simulink model "playback_data"  (R2015a)
settings: Solver=FixedStepDiscrete  SolverMode=SingleTasking  StartTime=76  StopTime=110  FixedStep=sample_time  RelTol=1e-3
undefined symbols (not defined in the file): A1_notch_f1, A2_notch_f1, A_kalman_swing_load, A_kalman_transverse, A_kalman_vertical, A_lpf_accelerometer, A_lpf_dtau, A_lpf_fourbar_angles, A_lpf_imu, A_lpf_lateral_angle, B1_lpf_accelerometer, B1_lpf_dtau, B1_lpf_fourbar_angles, B1_lpf_imu, B1_lpf_lateral_angle, B1_notch_f1, B2_lpf_accelerometer, B2_lpf_dtau, B2_lpf_fourbar_angles, B2_lpf_imu, B2_lpf_lateral_angle, B2_notch_f1, B_dx_versus_x0, B_kalman_swing_load, B_kalman_transverse, B_kalman_vertical, backwards_K_sag_of_t, backwards_P_sag_of_t, C_kalman_swing_load, C_kalman_transverse, C_kalman_vertical, com_leg_motor, com_torso, contact_threshold, control_start_time, d_ankle_to_foot, d_vertical_com, desired_com_forward_velocity, desired_com_lateral_velocity, desired_initial_leg_roll_left, desired_initial_leg_roll_right, desired_stance_beta2, desired_standing_torso_pitch, desired_standing_torso_roll, desired_standing_z, desired_torso_pitch, desired_torso_roll, Discrete, enable_bouncing, fcut_contact, fdesignblkfcn, forward_dx_of_dxstar, forward_x_of_dxstar, g, gcbh, HIP_MTR_MAX_CONT_TORQUE, HIP_MTR_MAX_TORQUE, i_leg_motor, i_robot, i_torso ... (+78)
libraries: simulink x65, dsparch4 x18, ctrlSharedLib x14, dspfdesign x4
(part 1 of 13)
settings Model: CovSFcnEnable=off  Creator=wmartin  LastModifiedBy=wmartin
settings SolverCC: EnableConcurrentExecution=on
settings DataIOCC: LimitDataPoints=off  MaxDataPoints=1000000000  SaveFormat=StructureWithTime  SignalLogging=off  DSMLogging=off  VisualizeSimOutput=off
settings OptimizationCC: BlockReduction=off  OptimizeBlockIOStorage=off  BufferReuse=off  GlobalBufferReuse=off  ExpressionFolding=off  ExpressionDepthLimit=2147483647  LocalBlockOutputs=off  SimCompilerOptimization=on
settings DebuggingCC: UnderspecifiedInitializationDetection=Classic  MergeDetectMultiDrivingBlocksExec=none  SolverPrmCheckMsg=warning  StateNameClashWarn=warning
settings HardwareCC: ProdIntDivRoundTo=Zero  ProdEndianess=LittleEndian  ProdLongLongMode=on  ProdHWDeviceType=Generic->32-bit x86 compatible
settings ModelReferenceCC: UpdateModelReferenceTargets=IfOutOfDate  ModelReferenceNumInstancesAllowed=Single  ModelReferenceMinAlgLoopOccurrences=on
settings RTWCC: SystemTargetFile=slrt.tlc  TemplateMakefile=slrt_default_tmf  Description=Simulink Real-Time  RTWVerbose=off  RTWCompilerOptimization=on
settings CodeAppCC: MaxIdLength=256
settings TargetCC: CodeReplacementLibrary=XPC_BLAS  ParMdlRefBuildCompliant=on  ConcurrentExecutionCompliant=on  MatFileLogging=on  MATLABClassNameForMDSCustomization=xpcAperiodicCustomization

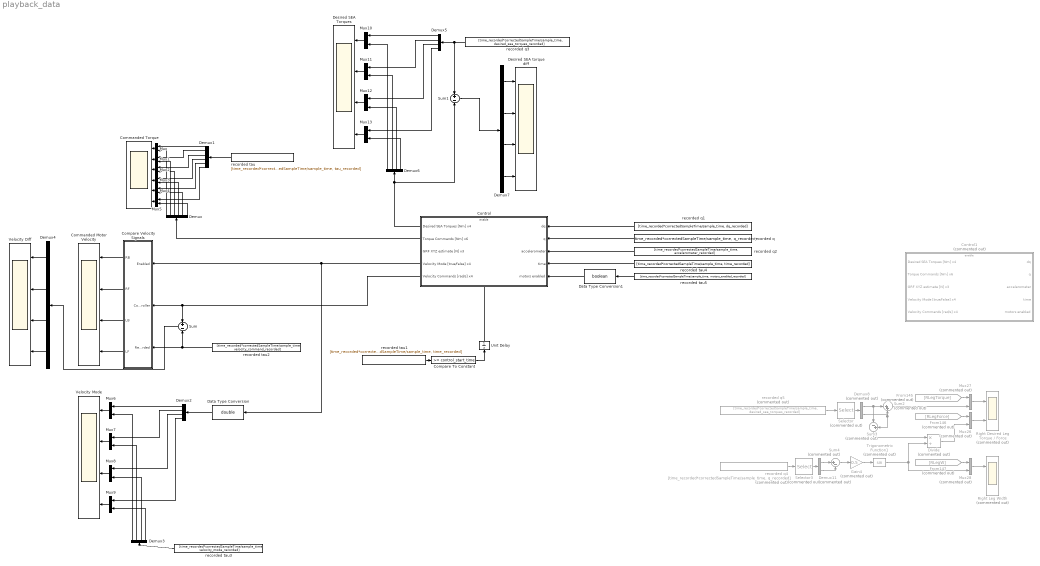
== system playback_data ==
  Commanded Motor Velocity : Scope  NumInputPorts=4
      settings: YMin=-0.45~-1~-1~-1  YMax=0.35~1~1~1  SaveName=SeaTorques  SampleInput=on  SampleTime=sample_time
  Commanded Torque : Scope  NumInputPorts=6
      settings: TimeRange=75  YMin=-75~-150~31~-1~-1~12.5  YMax=125~50~44~1~1~37.5  SampleInput=on
  Compare To Constant : simulink/Logic and Bit Operations/Compare To Constant  relop=>=  const=control_start_time  OutDataTypeStr=boolean
  Compare Velocity Signals : Subsystem
  Control : Subsystem
  Control1 : Subsystem  Commented=on
  Data Type Conversion : DataTypeConversion  OutDataTypeStr=double
  Data Type Conversion1 : DataTypeConversion  OutDataTypeStr=boolean
  Demux : Demux  Outputs=6
  Demux1 : Demux  Outputs=6
  Demux11 : Demux  Commented=on  Outputs=2
  Demux{2..7} (6 alike) : Demux
  Demux8 : Demux  Commented=on  Outputs=2
  Desired SEA Torques : Scope  NumInputPorts=4
      settings: YMin=-1~-1~-225~0  YMax=1~1~0~225  SaveName=SeaTorques3  SampleInput=on  SampleTime=sample_time
  Desired SEA torque diff : Scope  NumInputPorts=4
      settings: TimeRange=17.014  YMin=-1~-1~-0.35~-0.35  YMax=1~1~0.35~0.35  SaveName=SeaTorques4  SampleInput=on
  Divide : Product  Commented=on  Inputs=*/
  From145 : From  Commented=on  GotoTag=RLegTorque
  From146 : From  Commented=on  GotoTag=RLegForce
  From147 : From  Commented=on  GotoTag=RLegW
  Gain4 : Gain  Commented=on  Gain=0.5
  Mux{,1..13} (14 alike) : Mux  Inputs=2
  Mux26 : Mux  Commented=on  Inputs=2
  Mux27 : Mux  Commented=on  Inputs=2
  Mux28 : Mux  Commented=on  Inputs=2
  Right Desired Leg Torque / Force : Scope  Commented=on  NumInputPorts=2
      settings: YMin=0~-150  YMax=90~850  SaveName=ScopeData25  SampleInput=on
  Right Leg Width : Scope  Commented=on  NumInputPorts=2
      settings: YMin=0.57~-1  YMax=0.7~1  SaveName=ScopeData26  SampleInput=on
  Selector : Selector  Commented=on  InputPortWidth=4  Indices=[1 2]
  Selector3 : Selector  Commented=on  InputPortWidth=13  Indices=[1 3]
  Sum : Sum  Inputs=+-
  Sum1 : Sum  Inputs=+-
  Sum2 : Sum  Commented=on  Inputs=|++
  Sum3 : Sum  Commented=on  Inputs=|-+
  Sum4 : Sum  Commented=on  Inputs=|+-
  Trigonometric Function1 : Trigonometry  Commented=on
  Unit Delay : UnitDelay  SampleTime=-1
  Velocity Diff : Scope  NumInputPorts=4
      settings: YMin=-2~-2.5~-3~-4  YMax=2~2.5~3.5~2.5  SaveName=SeaTorques2  SampleInput=on
  Velocity Mode : Scope  NumInputPorts=4
      settings: YMin=1~1~-1~-1  YMax=1~1~1~1  SaveName=SeaTorques1  SampleInput=on  SampleTime=sample_time
  recorded q : FromWorkspace  VariableName=[time_recorded*correctedSampleTime/sample_time, q_recorded]  OutDataTypeStr=double  SampleTime=sample_time  OutputAfterFinalValue=Holding final value
  recorded q1 : FromWorkspace  VariableName=[time_recorded*correctedSampleTime/sample_time, dq_recorded]  OutDataTypeStr=double  SampleTime=sample_time  OutputAfterFinalValue=Holding final value
  recorded q2 : FromWorkspace  VariableName=[time_recorded*correctedSampleTime/sample_time, accelerometer_recorded]  OutDataTypeStr=double  SampleTime=sample_time  OutputAfterFinalValue=Holding final value
  recorded q3 : FromWorkspace  VariableName=[time_recorded*correctedSampleTime/sample_time, desired_sea_torques_recorded]  OutDataTypeStr=double  SampleTime=sample_time  OutputAfterFinalValue=Holding final value
  recorded q4 : FromWorkspace  Commented=on  VariableName=[time_recorded*correctedSampleTime/sample_time, q_recorded]  OutDataTypeStr=double  SampleTime=sample_time  OutputAfterFinalValue=Holding final value
  recorded q5 : FromWorkspace  Commented=on  VariableName=[time_recorded*correctedSampleTime/sample_time, desired_sea_torques_recorded]  OutDataTypeStr=double  SampleTime=sample_time  OutputAfterFinalValue=Holding final value
  recorded tau : FromWorkspace  VariableName=[time_recorded*correctedSampleTime/sample_time, tau_recorded]  OutDataTypeStr=double  SampleTime=sample_time  Interpolate=off  OutputAfterFinalValue=Holding final value
  recorded tau1 : FromWorkspace  VariableName=[time_recorded*correctedSampleTime/sample_time, time_recorded]  OutDataTypeStr=double  SampleTime=sample_time  OutputAfterFinalValue=Holding final value
  recorded tau2 : FromWorkspace  VariableName=[time_recorded*correctedSampleTime/sample_time, velocity_command_recorded]  OutDataTypeStr=double  SampleTime=sample_time  Interpolate=off  OutputAfterFinalValue=Holding final value
  recorded tau3 : FromWorkspace  VariableName=[time_recorded*correctedSampleTime/sample_time, velocity_mode_recorded]  OutDataTypeStr=double  SampleTime=sample_time  Interpolate=off  OutputAfterFinalValue=Holding final value
  recorded tau4 : FromWorkspace  VariableName=[time_recorded*correctedSampleTime/sample_time, time_recorded]  OutDataTypeStr=double  SampleTime=sample_time  OutputAfterFinalValue=Holding final value
  recorded tau5 : FromWorkspace  VariableName=[time_recorded*correctedSampleTime/sample_time, motors_enabled_recorded]  OutDataTypeStr=double  SampleTime=sample_time  OutputAfterFinalValue=Holding final value
  wires:
  recorded tau1/1 -> Compare To Constant/1
  Compare To Constant/1 -> Unit Delay/1
  Unit Delay/1 -> Control/Enable
  Control/2(Torque Commands [Nm] x6) -> Demux/1
  recorded tau/1 -> Demux1/1
  Mux/1 -> Commanded Torque/1
  Mux1/1 -> Commanded Torque/2
  Mux2/1 -> Commanded Torque/3
  Mux3/1 -> Commanded Torque/4
  Mux4/1 -> Commanded Torque/5
  Mux5/1 -> Commanded Torque/6
  Demux1/1 -> Mux/1
  Demux/1 -> Mux/2
  Demux1/2 -> Mux1/1
  Demux1/3 -> Mux2/1
  Demux1/4 -> Mux3/1
  Demux1/5 -> Mux4/1
  Demux1/6 -> Mux5/1
  Demux/2 -> Mux1/2
  Demux/3 -> Mux2/2
  Demux/4 -> Mux3/2
  Demux/5 -> Mux4/2
  Demux/6 -> Mux5/2
  Compare Velocity Signals/1(RB) -> Commanded Motor Velocity/1
  Compare Velocity Signals/2(RF) -> Commanded Motor Velocity/2
  Compare Velocity Signals/3(LB) -> Commanded Motor Velocity/3
  Compare Velocity Signals/4(LF) -> Commanded Motor Velocity/4
  Control/4(Velocity Mode [true/false] x4) -> Data Type Conversion/1, Compare Velocity Signals/1(Enabled)
  recorded tau2/1 -> Sum/2, Compare Velocity Signals/3(Recorded)
  Mux6/1 -> Velocity Mode/1
  Mux7/1 -> Velocity Mode/2
  Mux8/1 -> Velocity Mode/3
  Mux9/1 -> Velocity Mode/4
  Demux2/2 -> Mux7/1
  Demux2/3 -> Mux8/1
  Demux2/4 -> Mux9/1
  recorded tau3/1 -> Demux3/1
  Demux3/1 -> Mux6/2
  Demux3/2 -> Mux7/2
  Demux3/3 -> Mux8/2
  Demux3/4 -> Mux9/2
  Data Type Conversion/1 -> Demux2/1
  Demux2/1 -> Mux6/1
  Control/5(Velocity Commands [rad/s] x4) -> Sum/1, Compare Velocity Signals/2(Controller)
  Sum/1 -> Demux4/1
  Demux4/4 -> Velocity Diff/4
  Demux4/3 -> Velocity Diff/3
  Demux4/2 -> Velocity Diff/2
  Demux4/1 -> Velocity Diff/1
  Mux10/1 -> Desired SEA Torques/1
  Mux11/1 -> Desired SEA Torques/2
  Mux12/1 -> Desired SEA Torques/3
  Mux13/1 -> Desired SEA Torques/4
  Demux5/2 -> Mux11/1
  Demux5/3 -> Mux12/1
  Demux5/4 -> Mux13/1
  Demux6/1 -> Mux10/2
  Demux6/2 -> Mux11/2
  Demux6/3 -> Mux12/2
  Demux6/4 -> Mux13/2
  recorded q3/1 -> Demux5/1, Sum1/1
  Demux5/1 -> Mux10/1
  Control/1(Desired SEA Torques [Nm] x4) -> Sum1/2, Demux6/1
  Demux7/3 -> Desired SEA torque diff/3
  Demux7/2 -> Desired SEA torque diff/2
  Demux7/1 -> Desired SEA torque diff/1
  Demux7/4 -> Desired SEA torque diff/4
  Sum1/1 -> Demux7/1
  recorded q5/1 -> Selector/1
  Selector/1 -> Demux8/1
  Demux8/1 -> Sum3/1, Sum2/1
  Demux8/2 -> Sum3/2, Sum2/2
  Sum2/1 -> Mux27/2
  Sum3/1 -> Divide/1
  Mux27/1 -> Right Desired Leg Torque / Force/1
  Mux26/1 -> Right Desired Leg Torque / Force/2
  From146/1 -> Mux26/1
  From145/1 -> Mux27/1
  recorded q4/1 -> Selector3/1
  Selector3/1 -> Demux11/1
  Demux11/1 -> Sum4/1
  Demux11/2 -> Sum4/2
  Sum4/1 -> Gain4/1
  Gain4/1 -> Trigonometric Function1/1
  Trigonometric Function1/1 -> Divide/2, Mux28/2
  Divide/1 -> Mux26/2
  Mux28/1 -> Right Leg Width/1
  From147/1 -> Mux28/1
  recorded q1/1 -> Control/1(dq)
  recorded q/1 -> Control/2(q)
  recorded q2/1 -> Control/3(accelerometer)
  recorded tau4/1 -> Control/4(time)
  Data Type Conversion1/1 -> Control/5(motors enabled)
  recorded tau5/1 -> Data Type Conversion1/1

== system playback_data/Compare Velocity Signals ==
  Enabled : Inport
  Controller : Inport  Port=2
  Recorded : Inport  Port=3
  Demux : Demux
  Demux1 : Demux
  Demux2 : Demux
  Mux{6..9} (4 alike) : Mux  Inputs=2
  Product{,1..3} (4 alike) : Product
  RB : Outport
  RF : Outport  Port=2
  LB : Outport  Port=3
  LF : Outport  Port=4
  wires:
  Demux/3 -> Mux8/1
  Demux/2 -> Mux7/1
  Demux1/1 -> Mux6/2
  Demux/1 -> Mux6/1
  Product/1 -> RB/1
  Demux/4 -> Mux9/1
  Mux6/1 -> Product/2
  Demux1/4 -> Mux9/2
  Mux7/1 -> Product1/2
  Mux9/1 -> Product3/2
  Recorded/1 -> Demux1/1
  Demux2/3 -> Product2/1
  Demux1/2 -> Mux7/2
  Controller/1 -> Demux/1
  Demux2/1 -> Product/1
  Product3/1 -> LF/1
  Product1/1 -> RF/1
  Product2/1 -> LB/1
  Mux8/1 -> Product2/2
  Demux1/3 -> Mux8/2
  Enabled/1 -> Demux2/1
  Demux2/4 -> Product3/1
  Demux2/2 -> Product1/1

== system playback_data/Control ==
  dq : Inport
  q : Inport  Port=2
  accelerometer : Inport  Port=3
  time : Inport  Port=4
  motors enabled : Inport  Port=5
  Enable : EnablePort  StatesWhenEnabling=reset  PropagateVarSize=During execution  ShowOutputPort=on
  Actuator Control : ModelReference  ModelNameDialog=actuator_control  SimulationMode=Normal  ModelReferenceVersion=1.1246  CopyOfModelName=actuator_control  DefaultDataLogging=on
  Actuator Control with Torque SEA commands : Subsystem  Commented=on
  Behavior Control : Subsystem
  Compute Body Frame Accelerations : Subsystem
  Detect Change : simulink/Logic and Bit Operations/Detect Change  vinit=0  InputProcessing=Inherited  OutDataTypeStr=boolean
  Filter Velocities : Subsystem
  Mux : Mux
  Desired SEA Torques [Nm] x4 : Outport  InitialOutput=[0 0 0 0]
  Torque Commands [Nm] x6 : Outport  Port=2  InitialOutput=[0 0 0 0 0 0]
  GRF XYZ estimate [N] x3 : Outport  Port=3  InitialOutput=[0 0 0]
  Velocity Mode [true/false] x4 : Outport  Port=4  InitialOutput=[false false false false]
  Velocity Commands [rad/s] x4 : Outport  Port=5  InitialOutput=[0 0 0 0]
  wires:
  q/1 -> Behavior Control/4(q), Actuator Control/6
  Actuator Control/1 -> Torque Commands [Nm] x6/1
  Behavior Control/4(GRF XYZ estimates [N N N]) -> GRF XYZ estimate [N] x3/1
  Filter Velocities/1(filtered dq) -> Behavior Control/3(dq)
  dq/1 -> Filter Velocities/1(raw dq), Actuator Control/7
  Actuator Control/2 -> Velocity Mode [true/false] x4/1
  Actuator Control/3 -> Velocity Commands [rad/s] x4/1
  accelerometer/1 -> Compute Body Frame Accelerations/1(accelerometer [g] x3)
  Compute Body Frame Accelerations/1(accelerations [m/s^2] x3) -> Behavior Control/2(Body XYZ Acceleration [m/s^2] x3)
  Enable/1 -> Behavior Control/1(Enabled [true/false])
  Actuator Control/4 -> Desired SEA Torques [Nm] x4/1
  Mux/1 -> Actuator Control/1
  motors enabled/1 -> Detect Change/1
  Detect Change/1 -> Mux/4, Mux/3, Mux/2, Mux/1
  time/1 -> Behavior Control/5(time), Actuator Control/5
  Behavior Control/3(Stance / Swing Control [1/0] x4) -> Actuator Control/4
  Behavior Control/2(Velocity Commands [rad/s] x4) -> Actuator Control/3
  Behavior Control/1(Torque Commands [Nm] x6) -> Actuator Control/2

== system playback_data/Control1 ==
  dq : Inport
  q : Inport  Port=2
  accelerometer : Inport  Port=3
  time : Inport  Port=4
  motors enabled : Inport  Port=5
  Enable : EnablePort  StatesWhenEnabling=reset  PropagateVarSize=During execution  ShowOutputPort=on
  Actuator Control : ModelReference  ModelNameDialog=actuator_control  SimulationMode=Normal  ModelReferenceVersion=1.1246  CopyOfModelName=actuator_control  DefaultDataLogging=on
  Actuator Control with Torque SEA commands : Subsystem  Commented=on
  Behavior Control : Subsystem
  Compute Body Frame Accelerations : Subsystem
  Detect Change : simulink/Logic and Bit Operations/Detect Change  vinit=0  InputProcessing=Inherited  OutDataTypeStr=boolean
  Filter Velocities : Subsystem
  Mux : Mux
  Desired SEA Torques [Nm] x4 : Outport  InitialOutput=[0 0 0 0]
  Torque Commands [Nm] x6 : Outport  Port=2  InitialOutput=[0 0 0 0 0 0]
  GRF XYZ estimate [N] x3 : Outport  Port=3  InitialOutput=[0 0 0]
  Velocity Mode [true/false] x4 : Outport  Port=4  InitialOutput=[false false false false]
  Velocity Commands [rad/s] x4 : Outport  Port=5  InitialOutput=[0 0 0 0]
  wires:
  q/1 -> Behavior Control/4(q), Actuator Control/6
  Actuator Control/1 -> Torque Commands [Nm] x6/1
  Behavior Control/4(GRF XYZ estimates [N N N]) -> GRF XYZ estimate [N] x3/1
  Filter Velocities/1(filtered dq) -> Behavior Control/3(dq)
  dq/1 -> Filter Velocities/1(raw dq), Actuator Control/7
  Actuator Control/2 -> Velocity Mode [true/false] x4/1
  Actuator Control/3 -> Velocity Commands [rad/s] x4/1
  accelerometer/1 -> Compute Body Frame Accelerations/1(accelerometer [g] x3)
  Compute Body Frame Accelerations/1(accelerations [m/s^2] x3) -> Behavior Control/2(Body XYZ Acceleration [m/s^2] x3)
  Enable/1 -> Behavior Control/1(Enabled [true/false])
  Actuator Control/4 -> Desired SEA Torques [Nm] x4/1
  Mux/1 -> Actuator Control/1
  motors enabled/1 -> Detect Change/1
  Detect Change/1 -> Mux/4, Mux/3, Mux/2, Mux/1
  time/1 -> Behavior Control/5(time), Actuator Control/5
  Behavior Control/3(Stance / Swing Control [1/0] x4) -> Actuator Control/4
  Behavior Control/2(Velocity Commands [rad/s] x4) -> Actuator Control/3
  Behavior Control/1(Torque Commands [Nm] x6) -> Actuator Control/2

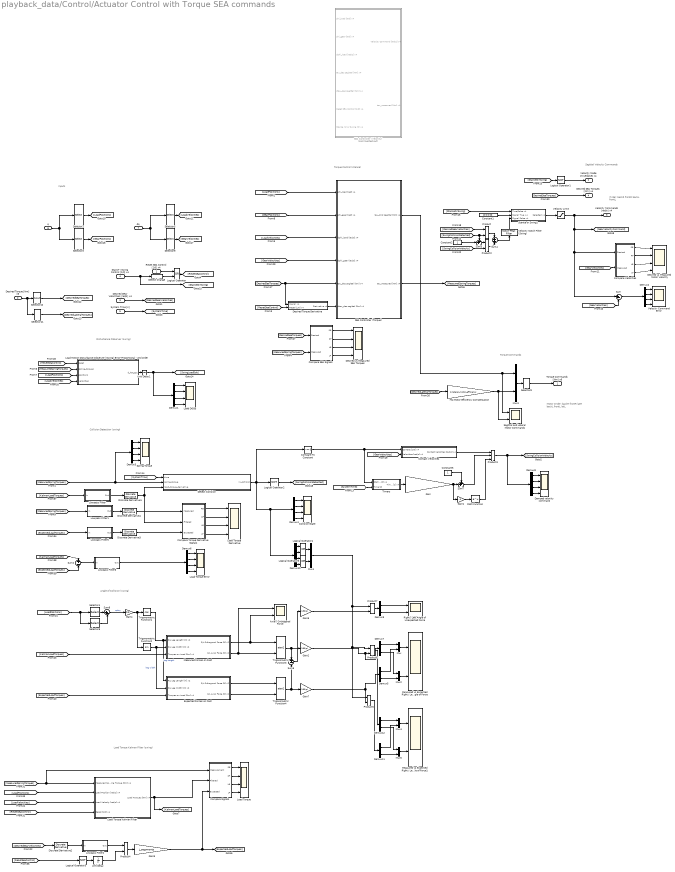
== system playback_data/Control/Actuator Control with Torque SEA commands ==
  note: Order:
      | backR
      | frontR
      | backL
      | frontL
  note: Motor Order:
      |
      | backR
      | frontR
      | latR
      | backL
      | frontL
      | latL
  note: Torque Control (stance)
  note: Inputs
  note: Disturbance Observer (swing)
  note: Torque Commands
  note: Sagittal Velocity Commands
  note: Collision Detection (swing)
  note: Load Torque Kalman Filter (swing)
  note: Angle of Collision (swing)
  Reset SEA Control [1/0] x4 : Inport  OutDataTypeStr=boolean  PortDimensions=4  SampleTime=sample_time
  Desired Torque [Nm] x6 : Inport  Port=2  OutDataTypeStr=double  PortDimensions=6  SampleTime=sample_time
  Desired Gear Velocities [rad/s] x4 : Inport  Port=3  OutDataTypeStr=double  PortDimensions=4  SampleTime=sample_time
  Stance / Swing Control [1/0] x4 : Inport  Port=4  OutDataTypeStr=boolean  PortDimensions=4  SampleTime=sample_time
  System Time [s] : Inport  Port=5  OutDataTypeStr=double  PortDimensions=1  SampleTime=sample_time
  q : Inport  Port=6  OutDataTypeStr=double  PortDimensions=13  SampleTime=sample_time
  dq : Inport  Port=7  OutDataTypeStr=double  PortDimensions=13  SampleTime=sample_time
  Axial / Orthogonal Force : Scope  NumInputPorts=2
      settings: YMin=-120~-175  YMax=120~150  SampleInput=on
  Collision State : Scope  NumInputPorts=4
      settings: YMin=0~-4~-1~-2.25  YMax=6~4~0.75~0  SaveName=LoadDOB_history2  SampleInput=on
  Compare To Constant : simulink/Logic and Bit Operations/Compare To Constant  relop=~=  const=0  OutDataTypeStr=boolean
  Compare SEA Signals : Subsystem
  Compare Signals : Subsystem
  Compare Torque Derivative Signals : Subsystem
  Compare Velocities : Subsystem
  Constant1 : Constant  Value=[0 0 0 0]
  Constant2 : Constant
  Constant5 : Constant
  Contact Velocities : Subsystem
  Damped velocity command : Scope  NumInputPorts=4
      settings: YMin=0~-4~-1~-2.25  YMax=6~4~0.75~0  SaveName=LoadDOB_history6  SampleInput=on
  Demux{1..4,6,8,10} (7 alike) : Demux
  Demux{5,7,9,11..12} (5 alike) : Demux  Outputs=2
  Desired Torque Derivative : Subsystem
  Desired vs Measured Motor Velocity : Scope  NumInputPorts=4
      settings: YMin=-0.03~-0.03~-0.025~-0.025  YMax=0.02~0.025~0.02~0.02  SaveName=ScopeData14  SampleInput=on
  Desired vs Measured SEA Torques : Scope  NumInputPorts=4
      settings: YMin=-35~-75~-500~-200  YMax=50~75~150~550  SaveName=SeaTorques  SampleInput=on  SampleTime=sample_time
  Detect Change : simulink/Logic and Bit Operations/Detect Change  vinit=0  InputProcessing=Inherited  OutDataTypeStr=boolean
  Detect Collision : MATLAB Function  TreatAsAtomicUnit=on
  Discrete Derivative{1..4} (4 alike) : simulink/Discrete/Discrete Derivative  gainval=1.0  ICPrevScaledInput=0.0  OutMin=[]  OutMax=[]  OutDataType=fixdt(1, 16)  OutScaling=2^-10  DoSatur=off
  Expected Forces on Foot : Subsystem
  Gain : Gain  Gain=swing_collision_damping_rate
  Gain1 : Gain  Gain=-1
  Gain2 : Gain  Gain=180/pi
  Gain4 : Gain  Gain=0.5
  Gain5 : Gain  Gain=j_segments
  Gain6 : Gain  Gain=180/pi
  Gain7 : Gain  Gain=180/pi
  Hip Motor Efficiency Compensation : Gain  Gain=1/lateral_motor_efficiency
  Load DOBs : Scope  NumInputPorts=4
      settings: YMin=-12~-7~2.7~-0.5  YMax=-8.75~1~4.1~2  SaveName=LoadDOB_history  SampleInput=on
  Load Motion Disturbance Observer (Swing) Error-Proportional - 2nd order : MATLAB Function  TreatAsAtomicUnit=on
  Load Torque : Scope  NumInputPorts=4
      settings: TimeRange=34.366  YMin=-300~-400~-100~-200  YMax=100~150~400~800  SaveName=LoadDOB_history3  SampleInput=on
  Load Torque Derivative : Scope  NumInputPorts=4
      settings: TimeRange=50.096  YMin=-4122.660296851378~-4185.660018993349~-3974.358974358969~-4680.851063829847  YMax=3871.203105284947~4522.792022792026~4743.58974358975~5531.914893616988  SaveName=LoadDOB_history4  SampleInput=on
  Load Torque Error : Scope  NumInputPorts=4
      settings: YMin=-100~-125~-125~-125  YMax=125~100~125~100  SaveName=LoadDOB_history5  SampleInput=on
  Load Torque Kalman Filter : Subsystem
  Logical Operator : Logic  Operator=OR  AllPortsSameDT=off  OutDataTypeStr=boolean
  Logical Operator1 : Logic  Operator=NOT  AllPortsSameDT=off  OutDataTypeStr=boolean
  Logical Operator2 : Logic  Operator=NOT  AllPortsSameDT=off  OutDataTypeStr=boolean
  Logical Operator3 : Logic  Operator=NOT  AllPortsSameDT=off  OutDataTypeStr=boolean
  Logical Operator4 : Logic  Operator=OR  AllPortsSameDT=off  OutDataTypeStr=boolean
  Logical Operator5 : Logic  Operator=OR  AllPortsSameDT=off  OutDataTypeStr=boolean
  Lowpass Filter : Subsystem  DialogController=fdesignblkfcn  InitFcn=fdesignblkfcn(gcbh, {'InitFcn'});  mask(Lowpass Filter){}
      mask help: Design a lowpass filter
      settings: CopyFcn=fdesignblkfcn(gcbh, {'CopyFcn'});
      mask Help: helpview(mapfilelocation('dsp'), 'dsplowpassfilter');
      mask Display: disp('Lowpass')
  Lowpass Filter1 : Subsystem  DialogController=fdesignblkfcn  InitFcn=fdesignblkfcn(gcbh, {'InitFcn'});  mask(Lowpass Filter){}
      mask help: Design a lowpass filter
      settings: CopyFcn=fdesignblkfcn(gcbh, {'CopyFcn'});
      mask Help: helpview(mapfilelocation('dsp'), 'dsplowpassfilter');
      mask Display: disp('Lowpass')
  Lowpass Filter2 : Subsystem  DialogController=fdesignblkfcn  InitFcn=fdesignblkfcn(gcbh, {'InitFcn'});  mask(Lowpass Filter){}
      mask help: Design a lowpass filter
      settings: CopyFcn=fdesignblkfcn(gcbh, {'CopyFcn'});
      mask Help: helpview(mapfilelocation('dsp'), 'dsplowpassfilter');
      mask Display: disp('Lowpass')
  Lowpass Filter5 : Subsystem  DialogController=fdesignblkfcn  InitFcn=fdesignblkfcn(gcbh, {'InitFcn'});  mask(Lowpass Filter){}
      mask help: Design a lowpass filter
      settings: CopyFcn=fdesignblkfcn(gcbh, {'CopyFcn'});
      mask Help: helpview(mapfilelocation('dsp'), 'dsplowpassfilter');
      mask Display: disp('Lowpass')
  Lowpass Filter6 : Subsystem  DialogController=fdesignblkfcn  InitFcn=fdesignblkfcn(gcbh, {'InitFcn'});  mask(Lowpass Filter){}
      mask help: Design a lowpass filter
      settings: CopyFcn=fdesignblkfcn(gcbh, {'CopyFcn'});
      mask Help: helpview(mapfilelocation('dsp'), 'dsplowpassfilter');
      mask Display: disp('Lowpass')
  Math Function : Math  SaturateOnIntegerOverflow=on
  Measured Forces on Foot : Subsystem
  Measured vs Expected Right / Left Angle of Force : Scope  NumInputPorts=2
      settings: TimeRange=45  YMin=-200~-200  YMax=200~200  SampleInput=on
  Measured vs Expected Right / Left Angle of Force1 : Scope  NumInputPorts=2
      settings: TimeRange=45  YMin=-1~-200  YMax=1~200  SaveName=ScopeData8  SampleInput=on
  Mux{,1..5} (6 alike) : Mux  Inputs=2
  Product{,2,4..7} (6 alike) : Product
  Product3 : Product  Inputs=3
  Right / Left Angle of Unexpected Force : Scope  NumInputPorts=2
      settings: TimeRange=45  YMin=-350~-400  YMax=300~350  SaveName=ScopeData3  SampleInput=on
  SEA Controller (Torque) : Subsystem
  SEA Controller (Velocity) : Subsystem  Commented=on
  Sagittal and Lateral Motor Commands : Scope  NumInputPorts=2
      settings: YMin=-1~0  YMax=1~65  SaveName=ScopeData2  SampleInput=on
  Selector1 : Selector  InputPortWidth=13  Indices=[1 3 5 7]
  Selector10 : Selector  InputPortWidth=6  Indices=[1 2 4 5]
  Selector11 : Selector  InputPortWidth=6  Indices=[3 6]
  Selector3 : Selector  InputPortWidth=13  Indices=[2 4 6 8]
  Selector4 : Selector  InputPortWidth=4  Indices=[1 3]
  Selector5 : Selector  InputPortWidth=13  Indices=[1 3 5 7]
  Selector6 : Selector  InputPortWidth=4  Indices=[2 4]
  Selector8 : Selector  InputPortWidth=6  Indices=[1 2 5 3 4 6]
  Selector9 : Selector  InputPortWidth=13  Indices=[2 4 6 8]
  Spring Torque : Scope  NumInputPorts=4
      settings: YMin=-75~-75~-75~-75  YMax=75~75~75~75  SaveName=LoadDOB_history1  SampleInput=on
  Stance or Swing1 : Subsystem
  Sum : Sum  Inputs=|+-
  Sum2 : Sum  Inputs=+|-
  Sum3 : Sum  Inputs=-+|
  Sum4 : Sum  Inputs=+|+
  Sum6 : Sum  Inputs=+|-
  Sum7 : Sum  Inputs=++|
  Sum8 : Sum  Inputs=|+-
  Timers : Subsystem
  Trigonometric Function1 : Trigonometry  Operator=cos
  Trigonometric Function2 : Trigonometry
  Trigonometric Function3 : Trigonometry  Operator=atan2
  Trigonometric Function4 : Trigonometry  Operator=atan2
  Unit Delay : UnitDelay  SampleTime=-1
  Unit Delay1 : UnitDelay  SampleTime=sample_time
  Velocity Command Error : Scope  NumInputPorts=4
      settings: YMin=-0.5~-0.4~-0.5~-1.5  YMax=1.5~0.5~0.9~0.75  SaveName=ScopeData6  SampleInput=on
  Velocity Limit : Saturate  UpperLimit=8  LowerLimit=-8
      settings: AttributesFormatString=Hi: %<UpperLimit>\nLo: %<LowerLimit>
  Velocity Notch Filter (Swing) : dspfdesign/Notch-Peak Filter  Specification=Quality factor and center frequency  Bandwidth=27  QualityFactor=2.5  CenterFrequency=27  BandwidthCoefficient=0.72654  CenterFrequencyCoefficient=0  Output=Notch  InheritSampleRate=off  SampleRate=update_freq  SimulateUsing=Code generation
  Torque Commands [Nm] x6 : Outport  OutDataTypeStr=double  PortDimensions=6  SampleTime=0  InitialOutput=[0 0 0 0 0 0]
  Velocity Mode [true/false] x4 : Outport  Port=2  InitialOutput=[false false false false]
  Velocity Commands [rad/s] x4 : Outport  Port=3  InitialOutput=[0 0 0 0]
  Desired SEA Torques [Nm] x4 : Outport  Port=4  InitialOutput=[false false false false]
  wires:
  Constant1/1 -> Stance or Swing1/2(Signal True x4)
  [StanceOrSwing] -> Logical Operator1/1
  [GearVelocities] -> SEA Controller (Torque)/4(dphi_gear [rad/s] x4)
  SEA Controller (Torque)/2(tau_measured [Nm] x4) -> [MeasuredSpringTorques]
  Selector8/1 -> Torque Commands [Nm] x6/1
  q/1 -> Selector1/1, Selector3/1
  [LoadPositions] -> SEA Controller (Torque)/1(phi_load [rad] x4)
  [DesiredSeaTorques] -> SEA Controller (Torque)/5(tau_des sagittal [Nm] x4), Desired Torque Derivative/1(Signal x4)
  [DesiredLateralTorques] -> Hip Motor Efficiency Compensation/1
  Mux3/1 -> Selector8/1
  Desired Torque Derivative/1(Derivative x4) -> SEA Controller (Torque)/6(dtau_des sagittal [Nm] x4)
  SEA Controller (Torque)/1(tau_cmd sagittal [Nm] x4) -> Sagittal and Lateral Motor Commands/1, Mux3/1
  Hip Motor Efficiency Compensation/1 -> Sagittal and Lateral Motor Commands/2, Mux3/2
  Compare SEA Signals/1(RB) -> Desired vs Measured SEA Torques/1
  Compare SEA Signals/2(RF) -> Desired vs Measured SEA Torques/2
  Compare SEA Signals/3(LB) -> Desired vs Measured SEA Torques/3
  Compare SEA Signals/4(LF) -> Desired vs Measured SEA Torques/4
  Compare Velocities/4(LF) -> Desired vs Measured Motor Velocity/4
  Compare Velocities/3(LB) -> Desired vs Measured Motor Velocity/3
  Compare Velocities/1(RB) -> Desired vs Measured Motor Velocity/1
  Compare Velocities/2(RF) -> Desired vs Measured Motor Velocity/2
  Load Motion Disturbance Observer (Swing) Error-Proportional - 2nd order/1(d_hat_tp1) -> Unit Delay1/1
  [MeasuredSpringTorques] -> Compare SEA Signals/2(Measured)
  [MeasuredSpringTorques] -> Load Motion Disturbance Observer (Swing) Error-Proportional - 2nd order/2(spring_torques)
  Selector1/1 -> [LoadPositions]
  Selector5/1 -> [LoadVelocities]
  [LoadPositions] -> Load Motion Disturbance Observer (Swing) Error-Proportional - 2nd order/3(positions)
  [LoadVelocities] -> Load Motion Disturbance Observer (Swing) Error-Proportional - 2nd order/4(velocities)
  Desired Torque [Nm] x6/1 -> Selector11/1, Selector10/1
  Selector11/1 -> [DesiredLateralTorques]
  [DesiredSeaTorques] -> Compare SEA Signals/1(Desired)
  [ResetSeaControl] -> Desired Torque Derivative/2(Reset [1/0] x4)
  [ResetSeaControl] -> Load Motion Disturbance Observer (Swing) Error-Proportional - 2nd order/1(reset)
  Logical Operator1/1 -> Velocity Mode [true/false] x4/1
  Demux1/1 -> Load DOBs/1
  Demux1/2 -> Load DOBs/2
  Demux1/3 -> Load DOBs/3
  Demux1/4 -> Load DOBs/4
  Unit Delay1/1 -> [SwingLoadDob], Demux1/1
  Stance / Swing Control [1/0] x4/1 -> [StanceOrSwing], Detect Change/1
  Logical Operator/1 -> [ResetSeaControl]
  Reset SEA Control [1/0] x4/1 -> Logical Operator/1
  [DesiredSeaTorques] -> Desired SEA Torques [Nm] x4/1
  [LoadVelocities] -> SEA Controller (Torque)/3(dphi_load [rad/s] x4)
  Selector3/1 -> [GearPositions]
  dq/1 -> Selector5/1, Selector9/1
  [GearPositions] -> SEA Controller (Torque)/2(phi_gear [rad] x4)
  [GearVelocities] -> Compare Velocities/2(Measured)
  [GearVelocities] -> Sum/2
  Sum/1 -> Demux2/1
  [DesiredGearVelocities] -> Product/1
  Demux2/4 -> Velocity Command Error/4
  Demux2/3 -> Velocity Command Error/3
  Demux2/2 -> Velocity Command Error/2
  Demux2/1 -> Velocity Command Error/1
  Demux3/4 -> Spring Torque/4
  Demux3/3 -> Spring Torque/3
  Demux3/2 -> Spring Torque/2
  Demux3/1 -> Spring Torque/1
  [SwingCollisionDetected] -> Sum3/1, Product/2
  Selector10/1 -> [DesiredSeaTorques]
  Constant2/1 -> Sum3/2
  [SwingCollisionVelocity] -> Product2/2
  Product/1 -> Sum4/1
  Product2/1 -> Sum4/2
  Sum3/1 -> Product2/1
  [KalmanLoadTorques] -> Lowpass Filter/1(In)
  Detect Collision/1(in_collision) -> Compare To Constant/1, Demux10/1, Demux4/1, Logical Operator2/1
  Stance or Swing1/1(Selected x4) -> Velocity Limit/1
  [StanceOrSwing] -> Stance or Swing1/1(True/False x4)
  Detect Change/1 -> Logical Operator/2
  Desired Gear Velocities [rad/s] x4/1 -> [DesiredGearVelocities]
  [GearVelocities] -> Contact Velocities/2(Velocities [rad/s] x4)
  Contact Velocities/1(Contact Velocities [rad/s] x4) -> Product3/1
  Compare To Constant/1 -> Contact Velocities/1(Contact [1/0] x4), Timers/1(Start [1/0] x4)
  Timers/1(Timer [s] x4) -> Gain/1
  Gain/1 -> Gain1/1, Sum7/2
  Constant5/1 -> Sum7/1
  Gain1/1 -> Math Function/1
  Math Function/1 -> Product3/3
  Product3/1 -> [SwingCollisionVelocity], Demux8/1
  Demux8/3 -> Damped velocity command/3
  Demux8/2 -> Damped velocity command/2
  Demux8/1 -> Damped velocity command/1
  Demux8/4 -> Damped velocity command/4
  [SystemTime] -> Timers/2(Time [s])
  Sum4/1 -> Velocity Notch Filter (Swing)/1
  Selector9/1 -> [GearVelocities]
  System Time [s]/1 -> [SystemTime]
  [SystemTime] -> Detect Collision/1(time)
  Demux4/3 -> Collision State/3
  Demux4/2 -> Collision State/2
  Demux4/1 -> Collision State/1
  Demux4/4 -> Collision State/4
  Logical Operator2/1 -> [SwingCollisionDetected]
  Selector4/1 -> Sum8/1
  Sum8/1 -> Gain4/1  "splay"
  Gain4/1 -> Trigonometric Function2/1, Trigonometric Function1/1
  [LoadPositions] -> Selector6/1, Selector4/1
  Demux7/2 -> Mux2/1
  Demux7/1 -> Mux/1
  [LoadVelocities] -> Load Torque Kalman Filter/3(Load Velocity [rad/s] x4)
  [ResetSeaControl] -> Load Torque Kalman Filter/4(Reset [1/0] x4)
  Compare Signals/3(LB) -> Load Torque/3
  Compare Signals/2(RF) -> Load Torque/2
  Compare Signals/4(LF) -> Load Torque/4
  Compare Signals/1(RB) -> Load Torque/1
  Load Torque Kalman Filter/1(Load Torques [Nm] x4) -> [KalmanLoadTorques], Compare Signals/2(Filtered)
  [MeasuredSpringTorques] -> Compare Signals/1(Measurement), Load Torque Kalman Filter/1(Measured Spring Torque [Nm] x4)
  [LoadPositions] -> Load Torque Kalman Filter/2(Load Position [rad/s] x4)
  Trigonometric Function3/1 -> Sum6/1, Gain2/1
  Product4/1 -> Gain5/1
  Gain5/1 -> [ExpectedLoadTorques], Compare Signals/3(Expected)
  Discrete Derivative2/1 -> Lowpass Filter2/1(In)
  Logical Operator3/1 -> Unit Delay/1
  [ResetSeaControl] -> Logical Operator3/1
  Unit Delay/1 -> Product4/2
  [ExpectedLoadTorques] -> Lowpass Filter5/1(In)
  Lowpass Filter5/1(Out) -> Discrete Derivative3/1
  Compare Torque Derivative Signals/4(LF) -> Load Torque Derivative/4
  Compare Torque Derivative Signals/3(LB) -> Load Torque Derivative/3
  Compare Torque Derivative Signals/2(RF) -> Load Torque Derivative/2
  Compare Torque Derivative Signals/1(RB) -> Load Torque Derivative/1
  [MeasuredSpringTorques] -> Lowpass Filter1/1(In)
  Lowpass Filter1/1(Out) -> Discrete Derivative4/1
  Discrete Derivative4/1 -> Compare Torque Derivative Signals/1(Measured)
  Demux6/3 -> Load Torque Error/3
  Demux6/2 -> Load Torque Error/2
  Demux6/1 -> Load Torque Error/1
  Demux6/4 -> Load Torque Error/4
  [KalmanLoadTorques] -> Sum2/1
  [ExpectedLoadTorques] -> Sum2/2
  Sum2/1 -> Lowpass Filter6/1(In)
  [DesiredGearVelocities] -> Discrete Derivative2/1
  Discrete Derivative3/1 -> Compare Torque Derivative Signals/3(Expected)
  Selector6/1 -> Sum8/2
  Demux5/2 -> Mux2/2
  Demux5/1 -> Mux/2
  Demux10/1 -> Logical Operator4/1
  Demux10/2 -> Logical Operator4/2
  Demux10/4 -> Logical Operator5/2
  Demux10/3 -> Logical Operator5/1
  Logical Operator4/1 -> Mux1/1
  Logical Operator5/1 -> Mux1/2
  Sum7/1 -> Product3/2
  Discrete Derivative1/1 -> Compare Torque Derivative Signals/2(Filtered), Detect Collision/3(load_torque_derivative)
  Lowpass Filter6/1(Out) -> Demux6/1
  Lowpass Filter/1(Out) -> Discrete Derivative1/1
  Lowpass Filter2/1(Out) -> Product4/1
  Trigonometric Function1/1 -> Expected Forces on Foot/1(R/L Leg Length [m] x2), Measured Forces on Foot/1(R/L Leg Length [m] x2)  "leg length"
  Trigonometric Function2/1 -> Measured Forces on Foot/2(R/L Leg Width [m] x2), Expected Forces on Foot/2(R/L Leg Width [m] x2)  "leg width"
  [KalmanLoadTorques] -> Measured Forces on Foot/3(Torques on Load [Nm] x4)
  Measured Forces on Foot/1(R/L Orthogonal Force [N] x2) -> Trigonometric Function3/1, Axial / Orthogonal Force/2
  Measured Forces on Foot/2(R/L Axial Force [N] x2) -> Axial / Orthogonal Force/1, Trigonometric Function3/2
  [ExpectedLoadTorques] -> Expected Forces on Foot/3(Torques on Load [Nm] x4)
  Expected Forces on Foot/1(R/L Orthogonal Force [N] x2) -> Trigonometric Function4/1
  Trigonometric Function4/1 -> Sum6/2, Gain7/1
  Gain6/1 -> Product7/2
  Demux9/1 -> Right / Left Angle of Unexpected Force/1
  Demux9/2 -> Right / Left Angle of Unexpected Force/2
  Expected Forces on Foot/2(R/L Axial Force [N] x2) -> Trigonometric Function4/2
  Mux2/1 -> Measured vs Expected Right / Left Angle of Force/2
  Mux/1 -> Measured vs Expected Right / Left Angle of Force/1
  Gain7/1 -> Demux5/1, Product5/2
  Gain2/1 -> Demux7/1, Product6/2
  Mux1/1 -> Product7/1, Product5/1, Product6/1
  Sum6/1 -> Gain6/1
  Product7/1 -> Demux9/1
  Demux12/2 -> Mux5/1
  Demux12/1 -> Mux4/1
  Demux11/2 -> Mux5/2
  Demux11/1 -> Mux4/2
  Mux5/1 -> Measured vs Expected Right / Left Angle of Force1/2
  Mux4/1 -> Measured vs Expected Right / Left Angle of Force1/1
  Product6/1 -> Demux12/1
  Product5/1 -> Demux11/1
  Velocity Notch Filter (Swing)/1 -> Stance or Swing1/3(Signal False x4)
  Velocity Limit/1 -> Velocity Commands [rad/s] x4/1, [GearVelocityCommand], Sum/1, Compare Velocities/1(Desired)
  [MeasuredSpringTorques] -> Demux3/1, Detect Collision/2(spring_torque)
